simulink model "mavsim_chap4"  (R2019a)
settings: Solver=ode45  StartTime=0.0  StopTime=10000  RelTol=1e-3  EnableMultiTasking=on
InitFcn:
  | param_chap4
undefined symbols (not defined in the file or in its folder): drawAircraft, forces_moments, P, plotmavstatevariables
libraries: simulink x4
settings Model: Creator=beard  LastModifiedBy=yuho8437
settings DataIOCC: LimitDataPoints=on  SaveFormat=Array  SignalLoggingSaveFormat=ModelDataLogs  ReturnWorkspaceOutputs=off
settings OptimizationCC: ExpressionDepthLimit=2147483647  InitFltsAndDblsToZero=on  LifeSpan=inf
settings DebuggingCC: UnderspecifiedInitializationDetection=Classic  MergeDetectMultiDrivingBlocksExec=none  SolverPrmCheckMsg=warning  FcnCallInpInsideContextMsg=warning  StateNameClashWarn=warning  SFUnexpectedBacktrackingDiag=warning  SFNoUnconditionalDefaultTransitionDiag=warning  SFExecutionAtInitializationDiag=none  ArithmeticOperatorsInVariantConditions=warning
settings HardwareCC: ProdBitPerPointer=32  ProdBitPerSizeT=32  ProdBitPerPtrDiffT=32  ProdLargestAtomicFloat=None  ProdIntDivRoundTo=Undefined  ProdEndianess=Unspecified  ProdWordSize=32  ProdHWDeviceType=32-bit Generic
settings ModelReferenceCC: PropagateSignalLabelsOutOfModel=off
settings SFSimCC: SimUseLocalCustomCode=off
settings RTWCC: RTWUseLocalCustomCode=off
settings CodeAppCC: StateflowObjectComments=on
settings GRTTargetCC: TargetLangStandard=C89/C90 (ANSI)  GeneratePreprocessorConditionals=Disable all  CombineOutputUpdateFcns=off  GRTInterface=on
settings ConfigComp: CovMetricSettings=dw  CovHtmlReporting=on  CovSaveCumulativeToWorkspaceVar=on  CovSaveSingleToWorkspaceVar=on  CovExternalEMLEnable=off  CovSFcnEnable=off

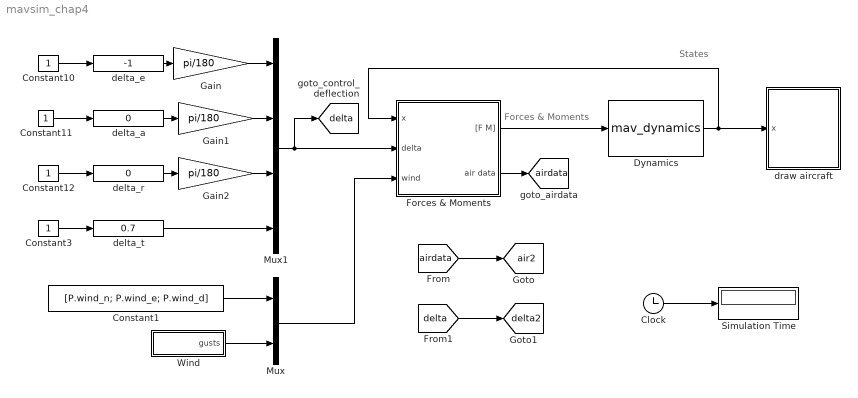
== system mavsim_chap4 ==
  note: Forces & Moments
  note: States
  Clock : Clock
  Constant1 : Constant  Value=[P.wind_n; P.wind_e; P.wind_d]
  Constant{3,10..12} (4 alike) : Constant
  Dynamics : S-Function  FunctionName=mav_dynamics  Parameters=P  SFunctionDeploymentMode=off  EnableBusSupport=off
  Forces & Moments : Subsystem
  Gain : Gain  Gain=pi/180
  Gain1 : Gain  Gain=pi/180
  Gain2 : Gain  Gain=pi/180
  Mux : Mux  Inputs=2
  Mux1 : Mux
  Simulation Time : Display
  Wind : Subsystem
  delta_a : simulink/Math Operations/Slider Gain  gain=0  low=-45  high=45
  delta_e : simulink/Math Operations/Slider Gain  gain=-1  low=-45  high=45
  delta_r : simulink/Math Operations/Slider Gain  gain=0  low=-45  high=45
  delta_t : simulink/Math Operations/Slider Gain  gain=0.7  low=0  high=1
  draw aircraft : Subsystem
      mask Display: image(imread('tv.jpg'))
  tag scope: air2=global, airdata=global, delta2=global, delta=global
  wires:
  Constant10/1 -> delta_e/1
  Constant11/1 -> delta_a/1
  Constant12/1 -> delta_r/1
  Dynamics/1 -> draw aircraft/1(x), Forces & Moments/1(x)
  delta_r/1 -> Gain2/1
  delta_a/1 -> Gain1/1
  delta_e/1 -> Gain/1
  Constant3/1 -> delta_t/1
  delta_t/1 -> Mux1/4
  Mux1/1 -> Forces & Moments/2(delta), [delta]
  Forces & Moments/1("[F M]") -> Dynamics/1
  Clock/1 -> Simulation Time/1
  Mux/1 -> Forces & Moments/3(wind)
  Wind/1(gusts) -> Mux/2
  Constant1/1 -> Mux/1
  Forces & Moments/2(air data) -> [airdata]
  Gain/1 -> Mux1/1
  Gain1/1 -> Mux1/2
  Gain2/1 -> Mux1/3
  [airdata] -> [air2]
  [delta] -> [delta2]

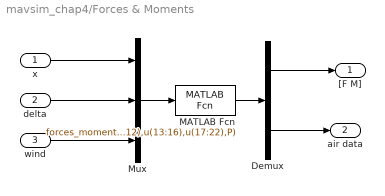
== system mavsim_chap4/Forces & Moments ==
  x : Inport
  delta : Inport  Port=2
  wind : Inport  Port=3
  Demux : Demux  Outputs=[6;6]
  MATLAB Fcn : MATLABFcn  MATLABFcn=forces_moments(u(1:12),u(13:16),u(17:22),P)  OutputDimensions=12
  Mux : Mux  Inputs=3
  "[F M]" : Outport
  air data : Outport  Port=2
  wires:
  x/1 -> Mux/1
  delta/1 -> Mux/2
  wind/1 -> Mux/3
  MATLAB Fcn/1 -> Demux/1
  Demux/1 -> "[F M]"/1
  Mux/1 -> MATLAB Fcn/1
  Demux/2 -> air data/1

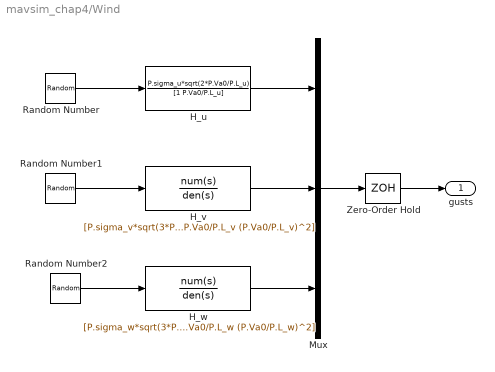
== system mavsim_chap4/Wind ==
  H_u : TransferFcn  Numerator=P.sigma_u*sqrt(2*P.Va0/P.L_u)  Denominator=[1 P.Va0/P.L_u]
  H_v : TransferFcn  Numerator=[P.sigma_v*sqrt(3*P.Va0/P.L_v) P.sigma_v*sqrt(3*P.Va0/P.L_v)*P.Va0/(sqrt(3)*P.L_v)]  Denominator=[1 2*P.Va0/P.L_v (P.Va0/P.L_v)^2]
  H_w : TransferFcn  Numerator=[P.sigma_w*sqrt(3*P.Va0/P.L_w) P.sigma_w*sqrt(3*P.Va0/P.L_w)*P.Va0/(sqrt(3)*P.L_w)]  Denominator=[1 2*P.Va0/P.L_w (P.Va0/P.L_w)^2]
  Mux : Mux  Inputs=3
  Random Number : RandomNumber  SampleTime=0
  Random Number1 : RandomNumber  SampleTime=0
  Random Number2 : RandomNumber  SampleTime=0
  Zero-Order Hold : ZeroOrderHold  SampleTime=P.Ts
  gusts : Outport
  wires:
  H_u/1 -> Mux/1
  Random Number/1 -> H_u/1
  Mux/1 -> Zero-Order Hold/1
  Zero-Order Hold/1 -> gusts/1
  Random Number1/1 -> H_v/1
  H_v/1 -> Mux/2
  Random Number2/1 -> H_w/1
  H_w/1 -> Mux/3

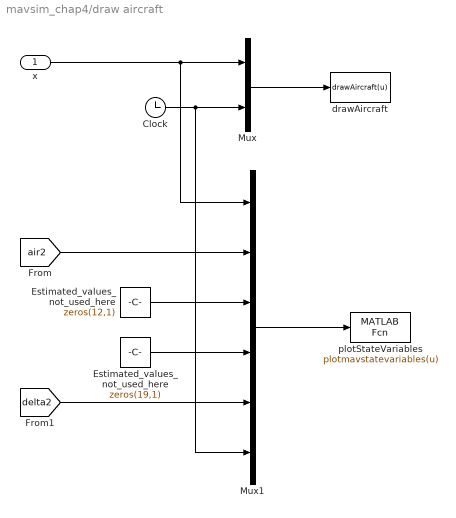
== system mavsim_chap4/draw aircraft ==
  x : Inport
  Clock : Clock
  Estimated_values_ not_used_here : Constant  Value=zeros(19,1)
  "Estimated_values_ not_used_here " : Constant  Value=zeros(12,1)
  Mux : Mux  Inputs=2
  Mux1 : Mux  Inputs=6
  drawAircraft : MATLABFcn  MATLABFcn=drawAircraft(u)  OutputDimensions=0  SampleTime=0.1
  plotStateVariables : MATLABFcn  MATLABFcn=plotmavstatevariables(u)  OutputDimensions=0  SampleTime=0.1
  wires:
  "Estimated_values_ not_used_here "/1 -> Mux1/3
  Estimated_values_ not_used_here/1 -> Mux1/4
  Mux1/1 -> plotStateVariables/1
  Clock/1 -> Mux1/6, Mux/2
  x/1 -> Mux1/1, Mux/1
  Mux/1 -> drawAircraft/1
  [air2] -> Mux1/2
  [delta2] -> Mux1/5
